simulink model "SimulacionControlR16"  (R2022b)
settings: Solver=VariableStepAuto  StartTime=0.0  StopTime=10  RelTol=1e-3
libraries: fuzblock x1
settings Model: Creator=PC-LUISMIGUEL  LastModifiedBy=PC-LUISMIGUEL

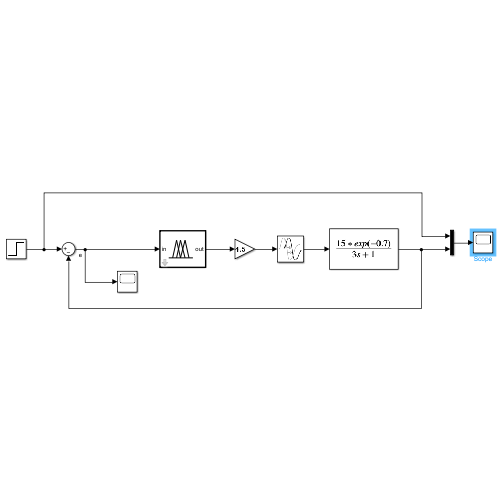
[thumbnail: Simulink's stored preview of the top-level diagram]
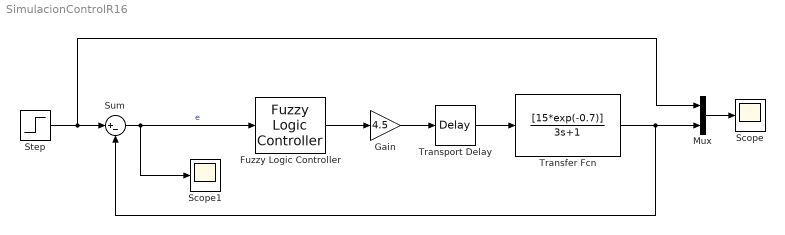
== system SimulacionControlR16 ==
  Fuzzy Logic Controller : fuzblock/Fuzzy Logic  Controller  FIS=Cdifuso  OutputSampleNumber=101  DataType=double  FuzzifiedInputs=off  RuleFiringStrengths=off  RuleOutputs=off  AggregatedOutputs=off  SimulateUsing=Interpreted execution  OutOfRangeInputValueMessage=warning  NoRuleFiredMessage=warning  EmptyOutputFuzzySetMessage=warning
  Gain : Gain  Gain=4.5
  Mux : Mux  Inputs=2
  Scope : Scope
  Scope1 : Scope
  Step : Step  Time=0  SampleTime=0
  Sum : Sum  Inputs=|+-
  Transfer Fcn : TransferFcn  Numerator=[15*exp(-0.7)]  Denominator=[3 1]
  Transport Delay : TransportDelay  DelayTime=0.7
  wires:
  Fuzzy Logic Controller/1 -> Gain/1
  Transfer Fcn/1 -> Mux/2, Sum/2
  Mux/1 -> Scope/1
  Gain/1 -> Transport Delay/1
  Transport Delay/1 -> Transfer Fcn/1
  Step/1 -> Mux/1, Sum/1
  Sum/1 -> Scope1/1, Fuzzy Logic Controller/1  "e"
